simulink model "Pendulum"  (R2023a)
settings: Solver=FixedStepAuto  StartTime=0.0  StopTime=10  FixedStep=0.01  RelTol=1e-3
settings Model: Creator=ZBW  LastModifiedBy=ZBW
settings SolverCC: AlgebraicLoopSolver=TrustRegion
settings DebuggingCC: UnconnectedInputMsg=warning  UnconnectedOutputMsg=warning  UnconnectedLineMsg=warning
settings ModelReferenceCC: EnableRefExpFcnMdlSchedulingChecks=on

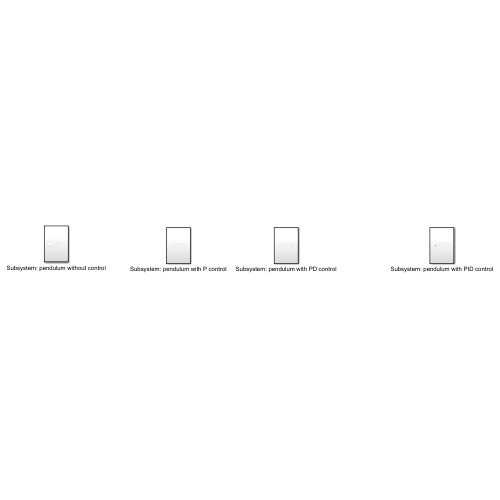
[thumbnail: Simulink's stored preview of the top-level diagram]
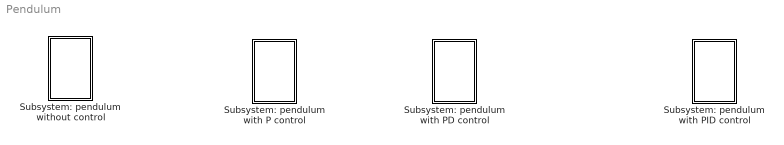
== system Pendulum ==
  Subsystem: pendulum with P control : Subsystem
  Subsystem: pendulum with PD control : Subsystem
  Subsystem: pendulum with PID control : Subsystem
  Subsystem: pendulum without control : Subsystem

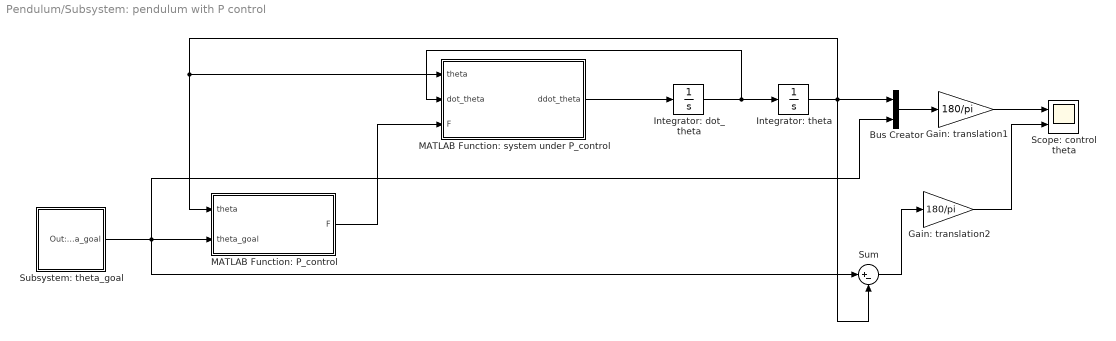
== system Pendulum/Subsystem: pendulum with P control ==
  Bus Creator : BusCreator  Inputs=2
  Gain: translation1 : Gain  Gain=180/pi
  Gain: translation2 : Gain  Gain=180/pi
  Integrator: dot_theta : Integrator
  Integrator: theta : Integrator  InitialCondition=pi/6
  MATLAB Function: P_control : MATLAB Function  TreatAsAtomicUnit=on
  MATLAB Function: system under P_control : MATLAB Function  TreatAsAtomicUnit=on
  Scope: control theta : Scope  NumInputPorts=2
  Subsystem: theta_goal : Subsystem
  Sum : Sum  Inputs=|+-
  wires:
  Integrator: dot_theta/1 -> MATLAB Function: system under P_control/2(dot_theta), Integrator: theta/1
  MATLAB Function: system under P_control/1(ddot_theta) -> Integrator: dot_theta/1
  MATLAB Function: P_control/1(F) -> MATLAB Function: system under P_control/3(F)
  Sum/1 -> Gain: translation2/1
  Integrator: theta/1 -> Bus Creator/1, MATLAB Function: P_control/1(theta), MATLAB Function: system under P_control/1(theta), Sum/2
  Subsystem: theta_goal/1(Out: theta_goal) -> Bus Creator/2, Sum/1, MATLAB Function: P_control/2(theta_goal)
  Bus Creator/1 -> Gain: translation1/1
  Gain: translation1/1 -> Scope: control theta/1
  Gain: translation2/1 -> Scope: control theta/2

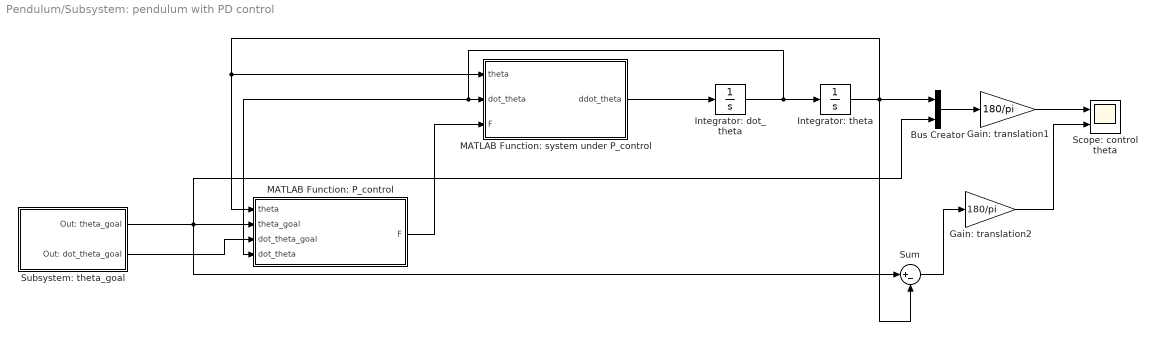
== system Pendulum/Subsystem: pendulum with PD control ==
  Bus Creator : BusCreator  Inputs=2
  Gain: translation1 : Gain  Gain=180/pi
  Gain: translation2 : Gain  Gain=180/pi
  Integrator: dot_theta : Integrator
  Integrator: theta : Integrator  InitialCondition=pi/6
  MATLAB Function: P_control : MATLAB Function  TreatAsAtomicUnit=on
  MATLAB Function: system under P_control : MATLAB Function  TreatAsAtomicUnit=on
  Scope: control theta : Scope  NumInputPorts=2
  Subsystem: theta_goal : Subsystem
  Sum : Sum  Inputs=|+-
  wires:
  Gain: translation2/1 -> Scope: control theta/2
  Gain: translation1/1 -> Scope: control theta/1
  Bus Creator/1 -> Gain: translation1/1
  Subsystem: theta_goal/1(Out: theta_goal) -> Sum/1, Bus Creator/2, MATLAB Function: P_control/2(theta_goal)
  Integrator: theta/1 -> Sum/2, MATLAB Function: system under P_control/1(theta), MATLAB Function: P_control/1(theta), Bus Creator/1
  Sum/1 -> Gain: translation2/1
  MATLAB Function: P_control/1(F) -> MATLAB Function: system under P_control/3(F)
  MATLAB Function: system under P_control/1(ddot_theta) -> Integrator: dot_theta/1
  Integrator: dot_theta/1 -> Integrator: theta/1, MATLAB Function: P_control/4(dot_theta), MATLAB Function: system under P_control/2(dot_theta)
  Subsystem: theta_goal/2(Out: dot_theta_goal) -> MATLAB Function: P_control/3(dot_theta_goal)

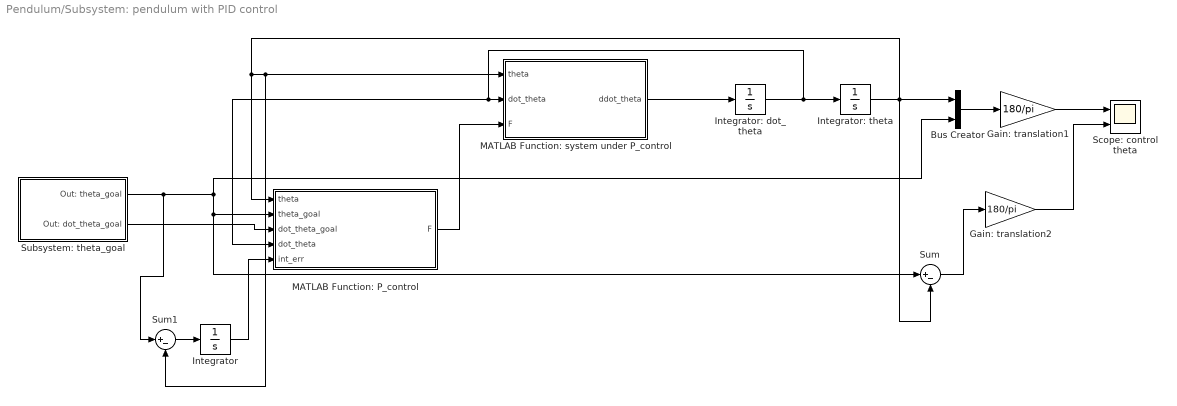
== system Pendulum/Subsystem: pendulum with PID control ==
  Bus Creator : BusCreator  Inputs=2
  Gain: translation1 : Gain  Gain=180/pi
  Gain: translation2 : Gain  Gain=180/pi
  Integrator : Integrator
  Integrator: dot_theta : Integrator
  Integrator: theta : Integrator  InitialCondition=pi/6
  MATLAB Function: P_control : MATLAB Function  TreatAsAtomicUnit=on
  MATLAB Function: system under P_control : MATLAB Function  TreatAsAtomicUnit=on
  Scope: control theta : Scope  NumInputPorts=2
  Subsystem: theta_goal : Subsystem
  Sum : Sum  Inputs=|+-
  Sum1 : Sum  Inputs=|+-
  wires:
  Subsystem: theta_goal/2(Out: dot_theta_goal) -> MATLAB Function: P_control/3(dot_theta_goal)
  Integrator: dot_theta/1 -> MATLAB Function: system under P_control/2(dot_theta), MATLAB Function: P_control/4(dot_theta), Integrator: theta/1
  MATLAB Function: system under P_control/1(ddot_theta) -> Integrator: dot_theta/1
  MATLAB Function: P_control/1(F) -> MATLAB Function: system under P_control/3(F)
  Sum/1 -> Gain: translation2/1
  Integrator: theta/1 -> Bus Creator/1, MATLAB Function: P_control/1(theta), MATLAB Function: system under P_control/1(theta), Sum1/2, Sum/2
  Subsystem: theta_goal/1(Out: theta_goal) -> Sum1/1, Sum/1, MATLAB Function: P_control/2(theta_goal), Bus Creator/2
  Bus Creator/1 -> Gain: translation1/1
  Gain: translation1/1 -> Scope: control theta/1
  Gain: translation2/1 -> Scope: control theta/2
  Sum1/1 -> Integrator/1
  Integrator/1 -> MATLAB Function: P_control/5(int_err)

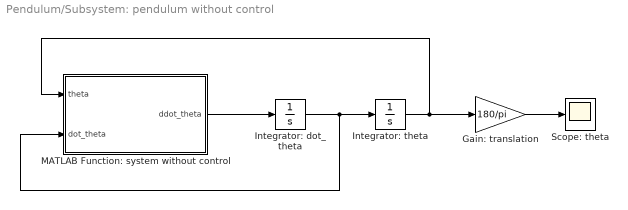
== system Pendulum/Subsystem: pendulum without control ==
  Gain: translation : Gain  Gain=180/pi
  Integrator: dot_theta : Integrator
  Integrator: theta : Integrator  InitialCondition=pi/6
  MATLAB Function: system without control : MATLAB Function  TreatAsAtomicUnit=on
  Scope: theta : Scope
  wires:
  MATLAB Function: system without control/1(ddot_theta) -> Integrator: dot_theta/1
  Integrator: dot_theta/1 -> MATLAB Function: system without control/2(dot_theta), Integrator: theta/1
  Integrator: theta/1 -> Gain: translation/1, MATLAB Function: system without control/1(theta)
  Gain: translation/1 -> Scope: theta/1

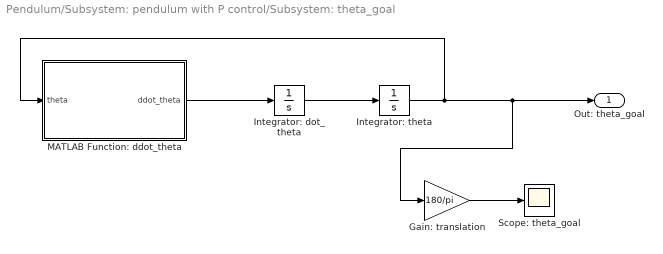
== system Pendulum/Subsystem: pendulum with P control/Subsystem: theta_goal ==
  Gain: translation : Gain  Gain=180/pi
  Integrator: dot_theta : Integrator
  Integrator: theta : Integrator  InitialCondition=pi/6
  MATLAB Function: ddot_theta : MATLAB Function  TreatAsAtomicUnit=on
  Scope: theta_goal : Scope
  Out: theta_goal : Outport
  wires:
  Integrator: dot_theta/1 -> Integrator: theta/1
  MATLAB Function: ddot_theta/1(ddot_theta) -> Integrator: dot_theta/1
  Integrator: theta/1 -> Gain: translation/1, Out: theta_goal/1, MATLAB Function: ddot_theta/1(theta)
  Gain: translation/1 -> Scope: theta_goal/1

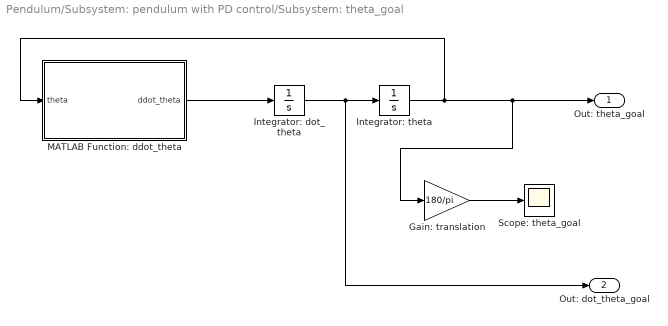
== system Pendulum/Subsystem: pendulum with PD control/Subsystem: theta_goal ==
  Gain: translation : Gain  Gain=180/pi
  Integrator: dot_theta : Integrator
  Integrator: theta : Integrator  InitialCondition=pi/3
  MATLAB Function: ddot_theta : MATLAB Function  TreatAsAtomicUnit=on
  Scope: theta_goal : Scope
  Out: theta_goal : Outport
  Out: dot_theta_goal : Outport  Port=2
  wires:
  Gain: translation/1 -> Scope: theta_goal/1
  Integrator: theta/1 -> MATLAB Function: ddot_theta/1(theta), Out: theta_goal/1, Gain: translation/1
  MATLAB Function: ddot_theta/1(ddot_theta) -> Integrator: dot_theta/1
  Integrator: dot_theta/1 -> Out: dot_theta_goal/1, Integrator: theta/1

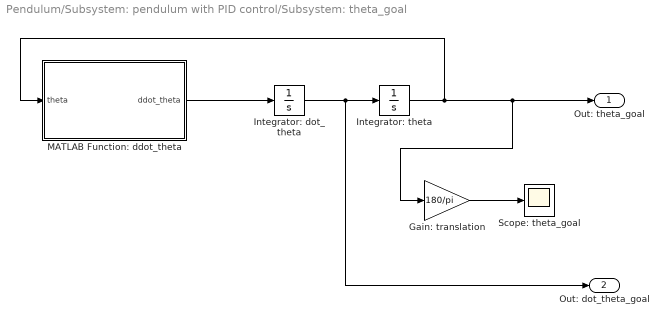
== system Pendulum/Subsystem: pendulum with PID control/Subsystem: theta_goal ==
  Gain: translation : Gain  Gain=180/pi
  Integrator: dot_theta : Integrator
  Integrator: theta : Integrator  InitialCondition=pi/7
  MATLAB Function: ddot_theta : MATLAB Function  TreatAsAtomicUnit=on
  Scope: theta_goal : Scope
  Out: theta_goal : Outport
  Out: dot_theta_goal : Outport  Port=2
  wires:
  Integrator: dot_theta/1 -> Integrator: theta/1, Out: dot_theta_goal/1
  MATLAB Function: ddot_theta/1(ddot_theta) -> Integrator: dot_theta/1
  Integrator: theta/1 -> Gain: translation/1, Out: theta_goal/1, MATLAB Function: ddot_theta/1(theta)
  Gain: translation/1 -> Scope: theta_goal/1

== matlab function Pendulum/Subsystem: pendulum with P control/Subsystem: theta_goal/MATLAB Function: ddot_theta ==
  data: theta input; ddot_theta output
function ddot_theta = fcn(theta)
g=9.81;
R=0.5;
ddot_theta = -g/R*theta;

== matlab function Pendulum/Subsystem: pendulum with P control/MATLAB Function: system under P_control ==
  data: theta input; ddot_theta output; dot_theta input; F input
function ddot_theta = fcn(theta,dot_theta,F)
g=9.81;
R=0.5;
c=0.1;
m=0.1;
ddot_theta = -g/R*theta-c/m*dot_theta+F/(m*R);

== matlab function Pendulum/Subsystem: pendulum with P control/MATLAB Function: P_control ==
  data: theta input; F output; theta_goal input
function F = fcn(theta,theta_goal)
kp=8;
F = (theta_goal-theta)*kp;

== matlab function Pendulum/Subsystem: pendulum without control/MATLAB Function: system without control ==
  data: theta input; ddot_theta output; dot_theta input
function ddot_theta = fcn(theta,dot_theta)
g=9.81;
R=0.5;
c=0.1;
m=0.1;
ddot_theta = -g/R*theta-c/m*dot_theta;

== matlab function Pendulum/Subsystem: pendulum with PD control/MATLAB Function: P_control ==
  data: theta input; F output; theta_goal input; dot_theta_goal input; dot_theta input
function F = fcn(theta,theta_goal,dot_theta_goal,dot_theta)
kp=2;
kd=0.5;
err=theta_goal-theta;
dot_err=dot_theta_goal-dot_theta;
F = err*kp+dot_err*kd;

== matlab function Pendulum/Subsystem: pendulum with PD control/MATLAB Function: system under P_control ==
  data: theta input; ddot_theta output; dot_theta input; F input
function ddot_theta = fcn(theta,dot_theta,F)
g=9.81;
R=0.5;
c=0.01;
m=0.1;
ddot_theta = -g/R*theta-c/m*dot_theta+F/(m*R);

== matlab function Pendulum/Subsystem: pendulum with PD control/Subsystem: theta_goal/MATLAB Function: ddot_theta ==
  data: theta input; ddot_theta output
function ddot_theta = fcn(theta)
g=9.81;
R=0.5;
ddot_theta = -g/R*theta;

== matlab function Pendulum/Subsystem: pendulum with PID control/MATLAB Function: P_control ==
  data: theta input; F output; theta_goal input; dot_theta_goal input; dot_theta input; int_err input
function F = fcn(theta,theta_goal,dot_theta_goal,dot_theta,int_err)
kp=8;
kd=1;
ki=5;
err=theta_goal-theta;
dot_err=dot_theta_goal-dot_theta;
F = err*kp+dot_err*kd+int_err*ki;

== matlab function Pendulum/Subsystem: pendulum with PID control/MATLAB Function: system under P_control ==
  data: theta input; ddot_theta output; dot_theta input; F input
function ddot_theta = fcn(theta,dot_theta,F)
g=9.81;
R=0.5;
c=0.01;
m=0.1;
dis=1;
ddot_theta = -g/R*theta-c/m*dot_theta+F/(m*R)+dis;

== matlab function Pendulum/Subsystem: pendulum with PID control/Subsystem: theta_goal/MATLAB Function: ddot_theta ==
  data: theta input; ddot_theta output
function ddot_theta = fcn(theta)
g=9.81;
R=0.5;
ddot_theta = -g/R*theta;
